simulink model "IEEE802153a_channel_model_test"  (Simulink 6.0)
settings: Solver=ode45  StartTime=0.0  StopTime=inf  RelTol=1e-3
libraries: dspsigattribs x4, dspsigops x3, dspbuff3 x2, dspmtrx3 x1, simulink x1
settings Model: LastModifiedBy=Robert
settings OptimizationCC: BlockReduction=off  BooleanDataType=off
settings DebuggingCC: SolverPrmCheckMsg=none
settings HardwareCC: TargetUnknown=on

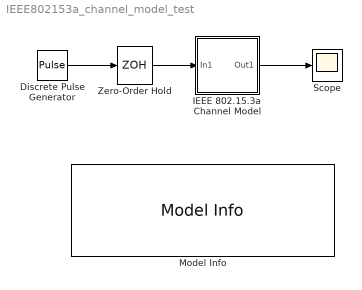
== system IEEE802153a_channel_model_test ==
  Discrete Pulse Generator : DiscretePulseGenerator  Period=5000  SampleTime=0.02e-9
  IEEE 802.15.3a Channel Model : Subsystem  Description=IEEE 802.15.3a channel model. It includes the four modes of the standard: CM1 through CM4, plus a custom setting  mask(IEEE Multipath Channel){T=0.02, nT=5000, SPF=2, chantype=CM3, LOSflag=off, LAMBDA=0.0667, lambda=2.1, GAMMA=14, gamma=7.9, sigma1=3.3941, sigma2=3.3941, std_shadow=3}
      mask prompts: T "Sample Time (nsec)"; nT "Symbol Period"; SPF "Symbols per Fade"; chantype "Channel Type"; LOSflag "LOS Channel"; sigma1 "sigma1 (dB)"; sigma2 "sigma2 (dB)"; std_shadow "Shadow sigma (dB)"
      mask help:
      | Filters the discrete-time input with a UWB channel realization.
      | Enter Sample Time in nsec.
      | Enter Symbol Period as a positive integer (number of sample times).
      | Enter Symbols per Fade as a positive integer to set duration over which the channel response is constant.
      | Choose a standard IEEE or Intel channel model, or enter custom parameters.
      mask init:
      | nTF = SPF * nT;
      mask Help:
      | The IEEE Multipath Channel block simulates an indoor UWB channel as described in "A Channel Model for Ultrawideband Indoor Communications" by J.R. Foerster, M. Pendergrass and A.F. Molisch, November 2003 and attempts to incorporate the processes used in their Matlab scripts.
      | 
      | The discrete input is convolved with a realization of the channel impulse response.  This response can be one of 4 types (CM1, CM2, CM3 or CM4) described in the paper or a custom channel with user-defined parameters.  A new channel realization is generated every symbol period.  Response terms that extend beyond one symbol period (ISI) are added to the output for the next symbol period.
      | 
      | Sample time is the rate at which the discrete signal is processed through the channel.  It represents the time resolution of the channel and is entered in nsec.  The symbol period is the time period of each data symbol and is entered as an integral number of sample times.  For example, enter
      | Sample Time:  0.02
      | Symbol Period:  100
      | for a signal with a symbol period of 2 nsec. and a sampling period of 20 psec.
      | 
      | Channel choices are
      | CM1             IEEE line of sight, < 4m
      | CM2             IEEE non-line of sight, < 4m
      | CM3             IEEE non-line of sight, 4-10m
      | CM4             IEEE strong dispersion, delay spread of 25 nsec.
      | custom         define parameters manually
      mask StyleString: edit,edit,edit,popup(CM1|CM2|CM3|CM4|Custom),checkbox,edit,edit,edit,edit,edit,edit,edit
      mask CallbackString: |||channel_maskcallback3||||||||
      mask Display:
      | plot([.1 .9],[0.1 0.1]);
      | plot([.1 .1],[0.1 .8]);
      | plot([.23 .23],[0.1 .35]);
      | plot([.3 .3],[0.1 .65]);
      | plot([.4 .4],[0.1 .2]);
      | plot([.55 .55],[0.1 0.3]);
      | plot([.7 .7],[0.1 .15]);
      | plot([.85 .85],[0.1 0.18]);
  Model Info : simulink/Model-Wide Utilities/Model Info  InitialBlockCM=none  BlockCM=none  Frame=on  DisplayStringWithTags=|  HorizontalTextAlignment=Center  LeftAlignmentValue=0.5  SourceBlockDiagram=IEEE802153a_channel_model_test  TagMaxNumber=20
      | IEEE 802.15.3a channel model
      | %<Created> by Tim Becker
      | Testbench Version %<ModelVersion> 
      | by Robert Morelos-Zaragoza
      | San Jose State University
      | Email: R.Morelos-Zaragoza@IEEE.org
  Scope : Scope
      settings: TimeRange=1e-007  YMin=-0.6  YMax=0.6
  Zero-Order Hold : ZeroOrderHold  SampleTime=0.02e-9
  wires:
  Discrete Pulse Generator/1 -> Zero-Order Hold/1
  Zero-Order Hold/1 -> IEEE 802.15.3a Channel Model/1(In1)
  IEEE 802.15.3a Channel Model/1(Out1) -> Scope/1

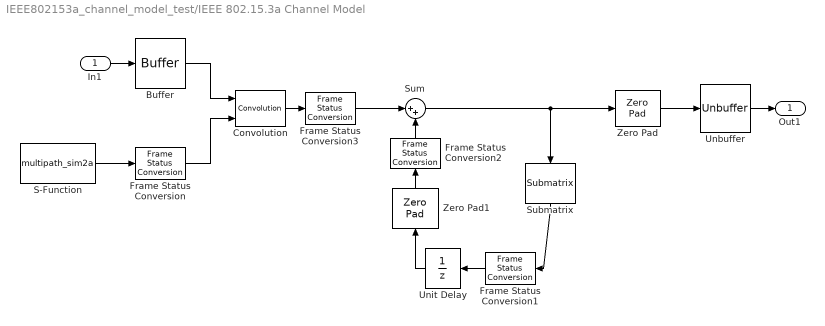
== system IEEE802153a_channel_model_test/IEEE 802.15.3a Channel Model ==
  In1 : Inport  Port=1  LatchInput=off
  Buffer : dspbuff3/Buffer  N=nT  V=0  ic=0
  Convolution : dspsigops/Convolution  DialogController=dspDDGCreate  DialogControllerArgs=DataTag0  domain=Time  roundingMode=Floor  overflowMode=off
  Frame Status Conversion : dspsigattribs/Frame Status Conversion  growRefPort=off  outframe=Frame-based
  Frame Status Conversion1 : dspsigattribs/Frame Status Conversion  Orientation=left  growRefPort=off  outframe=Sample-based
  Frame Status Conversion2 : dspsigattribs/Frame Status Conversion  Orientation=up  growRefPort=off  outframe=Frame-based
  Frame Status Conversion3 : dspsigattribs/Frame Status Conversion  growRefPort=off  outframe=Frame-based
  S-Function : S-Function  FunctionName=multipath_sim2a  Parameters=T,nTF,LAMBDA,lambda,GAMMA,gamma,sigma1,sigma2,std_shadow,LOSflag
  Submatrix : dspmtrx3/Submatrix  Orientation=down  RowSpan=Range of rows  RowStartMode=Index  RowStartIndex=nT+1  RowEndMode=Last  RowEndIndex=1  ColSpan=All columns  ColStartMode=First  ColStartIndex=1  ColEndMode=Last  ColEndIndex=1
  Sum : Sum  Inputs=|++  SaturateOnIntegerOverflow=on  InputSameDT=on
  Unbuffer : dspbuff3/Unbuffer  ic=0
  Unit Delay : UnitDelay  Orientation=left  SampleTime=nT*T*1e-9
  Zero Pad : dspsigops/Zero Pad  padSigAt=End  zpadAlong=Columns  padNumOutRowsSpecMethod=User-specified  numOutRows=nT  padNumOutColsSpecMethod=User-specified  numOutCols=1  trunc_flag=None
  Zero Pad1 : dspsigops/Zero Pad  Orientation=up  padSigAt=End  zpadAlong=Columns  padNumOutRowsSpecMethod=User-specified  numOutRows=10000+nT-1  padNumOutColsSpecMethod=User-specified  numOutCols=1  trunc_flag=None
  Out1 : Outport
  wires:
  S-Function/1 -> Frame Status Conversion/1
  Buffer/1 -> Convolution/1
  Frame Status Conversion/1 -> Convolution/2
  Zero Pad/1 -> Unbuffer/1
  Convolution/1 -> Frame Status Conversion3/1
  Sum/1 -> Zero Pad/1, Submatrix/1
  Submatrix/1 -> Frame Status Conversion1/1
  Frame Status Conversion1/1 -> Unit Delay/1
  Unit Delay/1 -> Zero Pad1/1
  Zero Pad1/1 -> Frame Status Conversion2/1
  Frame Status Conversion2/1 -> Sum/2
  In1/1 -> Buffer/1
  Unbuffer/1 -> Out1/1
  Frame Status Conversion3/1 -> Sum/1
